simulink model "spin_valto_Simulink"  (R2019b)
settings: Solver=ode45  StartTime=0.0  StopTime=0.000000025  FixedStep=1.0E-10  MaxStep=1.0E-10  RelTol=1.0E-5  AbsTol=1.0E-6
libraries: dspvision x1, dspmtrx3 x1
settings Model: Creator=krist  LastModifiedBy=krist
settings OptimizationCC: DefaultUnderspecifiedDataType=single

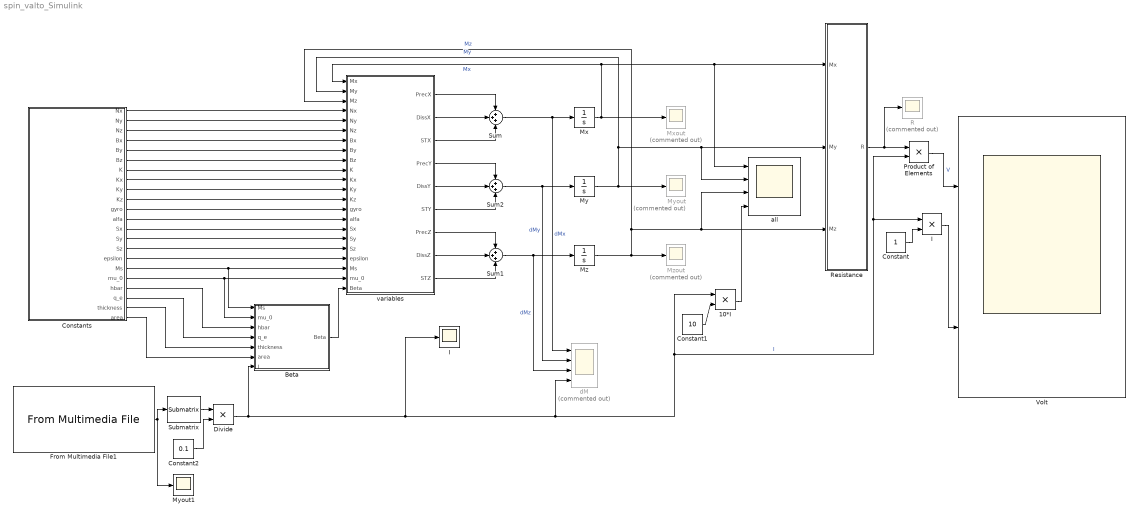
== system spin_valto_Simulink ==
  10*I : Product
  Beta : MATLAB Function  TreatAsAtomicUnit=on
  Constant : Constant
  Constant1 : Constant  Value=10
  Constant2 : Constant  Value=0.1
  Constants : MATLAB Function  TreatAsAtomicUnit=on
  Divide : Product
  From Multimedia File1 : dspvision/From Multimedia File  inputFilename=C:\Users\krist\OneDrive - hallgato.ppke.hu\AnitaSzakdolgozat\code\myrec\myrecordone3_rovid.wav  readRange=[1 Inf]  loop=on  numPlays=1  outputStreams=Audio only  videoDataType=single  audioDataType=double  inheritSampleTime=off  userDefinedSampleTime=1/6000000000  noAudioOutput=off  isIntensityVideo=off  fourcc=RGB  colorVideoFormat=Separate color signals  outputEOF=off  dataOrg=Column-major  audioFrameSize=16  computeAudioFrameSize=off  outSamplingMode=Sample based
      settings: SourceProductName=DSP System Toolbox  SourceProductBaseCode=DS
  I : Scope
  "I " : Product
  Mx : Integrator  InitialCondition=0.0706  AbsoluteTolerance=1.0E-6  IgnoreLimit=on
  Mxout : Scope  Commented=on
  My : Integrator  InitialCondition=0.9950  AbsoluteTolerance=1.0E-6  IgnoreLimit=on
  Myout : Scope  Commented=on
  Myout1 : Scope
  Mz : Integrator  InitialCondition=0.0707  AbsoluteTolerance=1.0E-6
  Mzout : Scope  Commented=on
  Product of Elements : Product
  R : Scope  Commented=on
  Resistance : MATLAB Function  TreatAsAtomicUnit=on
  Submatrix : dspmtrx3/Submatrix  RowSpan=One row  RowStartMode=Index  RowStartIndex=2  RowEndMode=Last  RowEndIndex=1  ColSpan=One column  ColStartMode=First  ColStartIndex=1  ColEndMode=Last  ColEndIndex=1
  Sum : Sum  Inputs=+++
  Sum1 : Sum  Inputs=+++
  Sum2 : Sum  Inputs=+++
  Volt : Scope  NumInputPorts=2
  all : Scope  NumInputPorts=4
  dM : Scope  Commented=on  NumInputPorts=4
  variables : MATLAB Function  TreatAsAtomicUnit=on
  wires:
  Beta/1(Beta) -> variables/22(Beta)
  Constants/19(hbar) -> Beta/3(hbar)
  Constants/20(q_e) -> Beta/4(q_e)
  Constants/21(thickness) -> Beta/5(thickness)
  Constants/22(area) -> Beta/6(area)
  Constants/1(Nx) -> variables/4(Nx)
  Constants/2(Ny) -> variables/5(Ny)
  Constants/3(Nz) -> variables/6(Nz)
  Constants/4(Bx) -> variables/7(Bx)
  Constants/5(By) -> variables/8(By)
  Constants/6(Bz) -> variables/9(Bz)
  Constants/7(K) -> variables/10(K)
  Constants/8(Kx) -> variables/11(Kx)
  Constants/9(Ky) -> variables/12(Ky)
  Constants/10(Kz) -> variables/13(Kz)
  Constants/11(gyro) -> variables/14(gyro)
  Constants/12(alfa) -> variables/15(alfa)
  Constants/13(Sx) -> variables/16(Sx)
  Constants/14(Sy) -> variables/17(Sy)
  Constants/15(Sz) -> variables/18(Sz)
  Constants/16(epsilon) -> variables/19(epsilon)
  variables/1(PrecX) -> Sum/1
  variables/4(PrecY) -> Sum2/1
  variables/7(PrecZ) -> Sum1/1
  variables/2(DissX) -> Sum/2
  variables/5(DissY) -> Sum2/2
  variables/8(DissZ) -> Sum1/2
  variables/3(STX) -> Sum/3
  variables/6(STY) -> Sum2/3
  variables/9(STZ) -> Sum1/3
  Mx/1 -> Mxout/1, Resistance/1(Mx), all/1, variables/1(Mx)  "Mx"
  Sum/1 -> dM/1, Mx/1  "dMx"
  My/1 -> Myout/1, all/2, Resistance/2(My), variables/2(My)  "My"
  Sum2/1 -> dM/2, My/1  "dMy"
  Mz/1 -> Mzout/1, variables/3(Mz), all/3, Resistance/3(Mz)  "Mz"
  Sum1/1 -> dM/3, Mz/1  "dMz"
  Resistance/1(R) -> Product of Elements/1, R/1
  Constants/17(Ms) -> variables/20(Ms), Beta/1(Ms)
  Constants/18(mu_0) -> variables/21(mu_0), Beta/2(mu_0)
  From Multimedia File1/1 -> Submatrix/1, Myout1/1
  Product of Elements/1 -> Volt/1  "V"
  Divide/1 -> I/1, dM/4, "I "/1, Product of Elements/2, 10*I/1, Beta/7(I)  "I"
  "I "/1 -> Volt/2
  Constant/1 -> "I "/2
  Constant1/1 -> 10*I/2
  10*I/1 -> all/4
  Constant2/1 -> Divide/2
  Submatrix/1 -> Divide/1

== matlab function spin_valto_Simulink/Beta ==
  data: Ms input; mu_0 input; hbar input; q_e input; thickness input; area input; I input; Beta output
function Beta  = fcn(Ms, mu_0, hbar, q_e, thickness, area, I)
%#codegen

Beta   = I * hbar / (mu_0*q_e*thickness*area*Ms);

== matlab function spin_valto_Simulink/Constants ==
  data: Nx output; Ny output; Nz output; Bx output; By output; Bz output; K output; Kx output; Ky output; Kz output; gyro output; alfa output; Sx output; Sy output; Sz output; epsilon output; Ms output; mu_0 output; hbar output; q_e output; thickness output; area output
function [Nx,Ny,Nz, Bx,By,Bz, K, Kx,Ky,Kz, gyro, alfa, Sx,Sy,Sz, epsilon, Ms, mu_0, hbar, q_e, thickness, area]= Constants
%#codegen
%The simulation time. Oscillations happen in the GHz range, so simulation
%time should be in the nanosecond range. 
Max_time = 20.0E-9;

%This is material parameter for permalloy (a widely used magnetic material)
%Leave this number unchanged
Ms = 8.6E+5;

%Further physical parameters. Leave them unchanged
gyro = 2.210E+5;
alfa =  0.01;   %This parameter must be fitted
hbar = 1.05457148E-34; 
mu_0 = 4*pi*1.0E-7;
q_e  = 1.60217646E-19; 

%These are parameters describing the geometry
%Nx + Ny + Nz = 1 must hold
%Nz > Nx, Nx=Ny describes a disc
%Use this as this is the simplest possible geometry
Nx = 0.0770;
Ny = 0.0770;
Nz = 0.8459;

K = 5.0E+5;

%This describes the current spin polarization
%Use these numbers for 
Sx = 1.0;
Sy = 0.0;
Sz = 0.0;

%Anisotropy axes
Kx = 0.0;
Ky = 0.0;
Kz = 1.0;

Bx = 0.001;
By = 0.001;
Bz = 0.5;

P           = 0.5; %Spin polarization
Lambda      = 1.5; %Spin-transfer parameter
thickness   = 5.0E-9;
area        = pi*(15.0E-9)^2;
Phi = 1.5;
Theta = 1.5;
Mxinit = cos(Phi)*sin(Theta);
Myinit = sin(Phi)*sin(Theta);
Mzinit = cos(Theta);
epsilon = (P*Lambda^2) / ( (Lambda^2+1) + (Lambda^2-1)*(Mxinit*Sx+Myinit*Sy+Mzinit*Sz) );

== matlab function spin_valto_Simulink/Resistance ==
  data: R output; Mx input; My input; Mz input
function R = Resistance(Mx, My, Mz)
%#codegen

R=Mx./sqrt(Mx.^2+My.^2+Mz.^2);

== matlab function spin_valto_Simulink/variables ==
  data: Mx input; My input; Mz input; Nx input; Ny input; Nz input; Bx input; By input; Bz input; K input; Kx input; Ky input; Kz input; gyro input; alfa input; Sx input; Sy input; Sz input; epsilon input; Ms input; mu_0 input; Beta input; PrecX output; DissX output; STX output; PrecY output; DissY output; STY output; PrecZ output; DissZ output; STZ output
function [PrecX,DissX,STX, PrecY,DissY,STY, PrecZ,DissZ,STZ]= variables(Mx,My,Mz, Nx,Ny,Nz, Bx,By,Bz, K, Kx,Ky,Kz, gyro, alfa, Sx,Sy,Sz, epsilon, Ms, mu_0, Beta)
%#codegen

Hx = -Nx*Mx*Ms + Bx/mu_0 + 2.0*K/(mu_0*Ms)*(Kx*Mx + Ky*My + Kz*Mz) * Kx;
Hy = -Ny*My*Ms + By/mu_0 + 2.0*K/(mu_0*Ms)*(Kx*Mx + Ky*My + Kz*Mz) * Ky;
Hz = -Nz*Mz*Ms + Bz/mu_0 + 2.0*K/(mu_0*Ms)*(Kx*Mx + Ky*My + Kz*Mz) * Kz;

PrecX = -gyro*( My*Hz - Mz*Hy );
PrecY = -gyro*( Mz*Hx - Mx*Hz );
PrecZ = -gyro*( Mx*Hy - My*Hx );

DissX = -alfa*gyro*( My*(Mx*Hy-My*Hx) - Mz*(Mz*Hx-Mx*Hz) );
DissY = -alfa*gyro*( Mz*(My*Hz-Mz*Hy)  - Mx*(Mx*Hy-My*Hx) );
DissZ = -alfa*gyro*( Mx*(Mz*Hx-Mx*Hz) - My*(My*Hz-Mz*Hy) );

STX   = gyro * Beta * epsilon * (My*(Sx*My-Sy*Mx) - Mz*(Sz*Mx-Sx*Mz));
STY   = gyro * Beta * epsilon * (Mz*(Sy*Mz-Sz*My) - Mx*(Sx*My-Sy*Mx));
STZ   = gyro * Beta * epsilon * (Mx*(Sz*Mx-Sx*Mz) - My*(Sy*Mz-Sz*My));
